simulink model "e102_digital_control_part7"  (R2024b)
settings: Solver=VariableStepAuto  StartTime=0.0  StopTime=10.0  RelTol=1e-3
values from neighbouring files (symbols this model uses):
  A = [-1/2, 1/2; 0, -2]    [E102_DC_RC_Part6.m]    (also in E102_DC_RC_Part_6_7_8.m)
  B = [0; 2]    [E102_DC_RC_Part6.m]    (also in E102_DC_RC_Part_6_7_8.m)
  C = [1, 0]    [E102_DC_RC_Part6.m]    (also in E102_DC_RC_Part_6_7_8.m)
  D = 0    [E102_DC_RC_Part6.m]    (also in E102_DC_RC_Part_6_7_8.m)
  Kr = 1 / (Cd * inv(eye(2) - (Ad - Bd*K)) * Bd)    [E102_DC_RC_Part6.m]    (also in E102_DC_RC_Part_6_7_8.m)
  L = place(Ad', Cd', poles_obsv)'    [E102_DC_RC_Part6.m]    (also in E102_DC_RC_Part_6_7_8.m)
undefined symbols (not defined in the file or in its folder): Ad, Bd, K
settings Model: Creator=sebastianheredia  LastModifiedBy=sebastianheredia

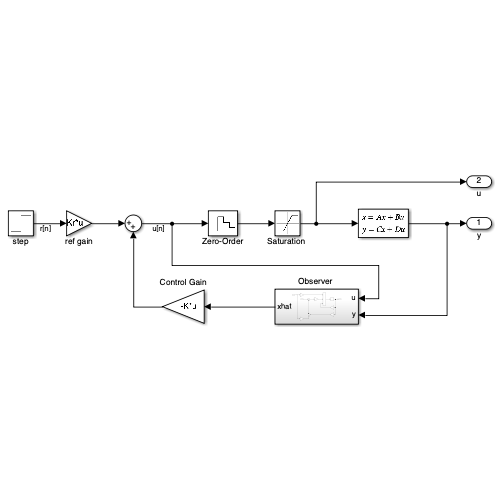
[thumbnail: Simulink's stored preview of the top-level diagram]
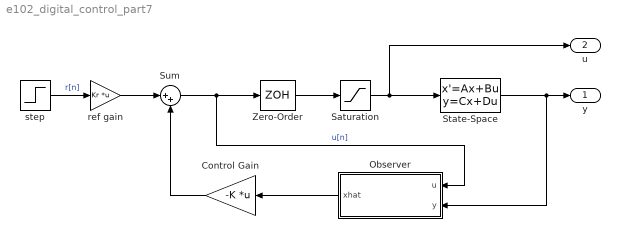
== system e102_digital_control_part7 ==
  Control Gain : Gain  Gain=-K  Multiplication=Matrix(K*u)
  "Observer " : Subsystem
  "Saturation " : Saturate  UpperLimit=5  LowerLimit=0
  State-Space : StateSpace  A=A  B=B  C=C  D=D  InitialCondition=0
  Sum : Sum  Inputs=|++
  Zero-Order : ZeroOrderHold  SampleTime=0.1
  ref gain : Gain  Gain=Kr  Multiplication=Matrix(K*u)
  step : Step  After=2.5  SampleTime=0
  y : Outport
  u : Outport  Port=2
  wires:
  step/1 -> ref gain/1  "r[n]"
  ref gain/1 -> Sum/1
  Sum/1 -> "Observer "/1(u), Zero-Order/1  "u[n]"
  Zero-Order/1 -> "Saturation "/1
  "Saturation "/1 -> State-Space/1, u/1
  Control Gain/1 -> Sum/2
  "Observer "/1(xhat) -> Control Gain/1
  State-Space/1 -> "Observer "/2(y), y/1

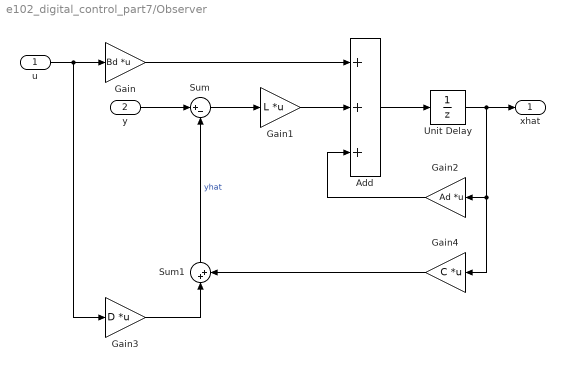
== system e102_digital_control_part7/Observer  ==
  u : Inport
  y : Inport  Port=2
  Add : Sum  Inputs=+++
  Gain : Gain  Gain=Bd  Multiplication=Matrix(K*u)
  Gain1 : Gain  Gain=L  Multiplication=Matrix(K*u)
  Gain2 : Gain  Gain=Ad  Multiplication=Matrix(K*u)
  Gain3 : Gain  Gain=D  Multiplication=Matrix(K*u)
  Gain4 : Gain  Gain=C  Multiplication=Matrix(K*u)
  Sum : Sum  Inputs=|+-
  Sum1 : Sum  Inputs=|++
  "Unit Delay " : UnitDelay  SampleTime=0.1  HasFrameUpgradeWarning=on
  xhat : Outport
  wires:
  u/1 -> Gain3/1, Gain/1
  y/1 -> Sum/1
  Sum/1 -> Gain1/1
  Gain/1 -> Add/1
  Gain1/1 -> Add/2
  Add/1 -> "Unit Delay "/1
  Gain2/1 -> Add/3
  Sum1/1 -> Sum/2  "yhat"
  Gain3/1 -> Sum1/1
  Gain4/1 -> Sum1/2
  "Unit Delay "/1 -> Gain4/1, Gain2/1, xhat/1
